simulink model "test"  (Simulink 7.7)
settings: Solver=ode45  StartTime=0.0  StopTime=10.0  RelTol=1e-3
settings Model: Creator=ISIT-Eric J.Huang  LastModifiedBy=ISIT-Eric J.Huang

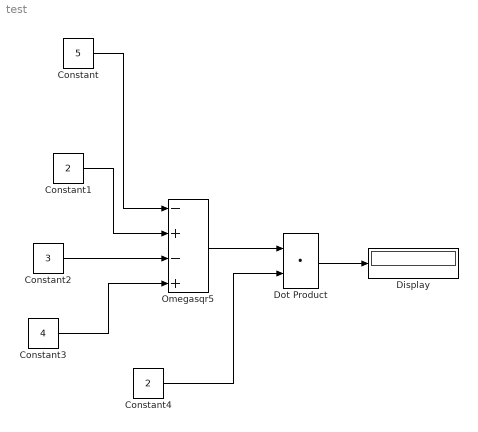
== system test ==
  Constant : Constant  Value=5
  Constant1 : Constant  Value=2
  Constant2 : Constant  Value=3
  Constant3 : Constant  Value=4
  Constant4 : Constant  Value=2
  Display : Display
  Dot Product : DotProduct  InputSameDT=on  OutDataTypeStr=Inherit: Inherit via internal rule
  Omegasqr5 : Sum  Inputs=-+-+
  wires:
  Omegasqr5/1 -> Dot Product/1
  Constant4/1 -> Dot Product/2
  Dot Product/1 -> Display/1
  Constant/1 -> Omegasqr5/1
  Constant1/1 -> Omegasqr5/2
  Constant2/1 -> Omegasqr5/3
  Constant3/1 -> Omegasqr5/4
